simulink model "Mounna_FrottementsNew"  (R2025b)
settings: Solver=ode45  StartTime=0.0  StopTime=TimeTqStop  MaxStep=0.1  RelTol=1e-3  EnableMultiTasking=on
undefined symbols (not defined in the file): Kv, RegimeTq, TempsTq, TorqueLosesTest, TorqueLosesTimeTest
settings Model: Creator=a030141  LastModifiedBy=Etudiant
settings SolverCC: AlgebraicLoopSolver=TrustRegion
settings DataIOCC: LimitDataPoints=on  SaveFormat=Array  SignalLoggingSaveFormat=ModelDataLogs  ReturnWorkspaceOutputs=off  SignalLoggingName=sigsOut
settings OptimizationCC: InitFltsAndDblsToZero=on  LifeSpan=inf
settings DebuggingCC: SaveWithParameterizedLinksMsg=none  UnderspecifiedInitializationDetection=Classic  MergeDetectMultiDrivingBlocksExec=none  SignalResolutionControl=TryResolveAllWithWarning  MultiTaskDSMMsg=warning  MultiTaskCondExecSysMsg=none  FcnCallInpInsideContextMsg=warning  UnconnectedInputMsg=warning  UnconnectedOutputMsg=warning  UnconnectedLineMsg=warning  SFUnexpectedBacktrackingDiag=warning  SFNoUnconditionalDefaultTransitionDiag=warning  SFExecutionAtInitializationDiag=none  ArithmeticOperatorsInVariantConditions=warning
settings HardwareCC: ProdBitPerPointer=32.0  ProdBitPerSizeT=32.0  ProdBitPerPtrDiffT=32.0  ProdLargestAtomicFloat=None  ProdIntDivRoundTo=Undefined  ProdEndianess=Unspecified  ProdWordSize=32.0  ProdHWDeviceType=32-bit Generic  TargetUnknown=on
settings ModelReferenceCC: PropagateSignalLabelsOutOfModel=off
settings RTWCC: GPUComputeCapability=3.5
settings CodeAppCC: StateflowObjectComments=on
settings GRTTargetCC: TargetFcnLib=ansi_tfl_tmw.mat  TargetLangStandard=C89/C90 (ANSI)  CombineOutputUpdateFcns=off  GRTInterface=on
settings ConfigComp: CovMetricSettings=dw  CovSaveCumulativeToWorkspaceVar=on  CovSaveSingleToWorkspaceVar=on

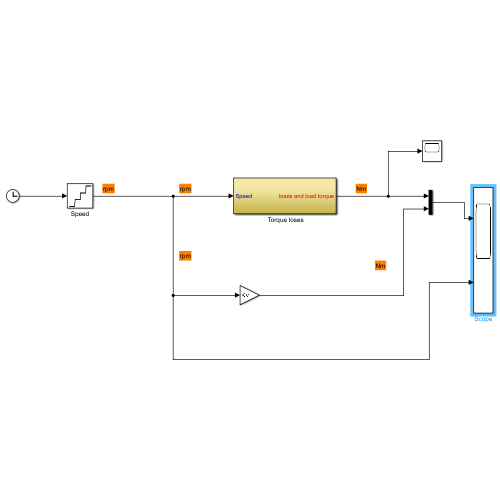
[thumbnail: Simulink's stored preview of the top-level diagram]
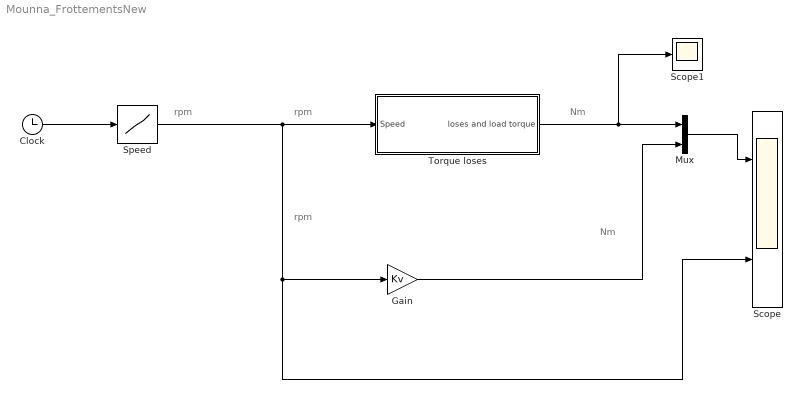
== system Mounna_FrottementsNew ==
  note: Nm
  note: rpm
  note: rpm
  note: rpm
  note: Nm
  " Torque loses" : Subsystem
  Clock : Clock
  Gain : Gain  Gain=Kv
  Mux : Mux  Inputs=2
  Scope : Scope  NumInputPorts=2
      settings: Title=Couple [Nm]  ActiveDisplayYMinimum=-114.2769674671385  ActiveDisplayYMaximum=10.919663051904275
  Scope1 : Scope
      settings: ActiveDisplayYMinimum=-1  ActiveDisplayYMaximum=1
  Speed : Lookup  InputValues=TempsTq  Table=RegimeTq
  wires:
  Clock/1 -> Speed/1
  Speed/1 -> Scope/2, Gain/1, " Torque loses"/1(Speed)
  Mux/1 -> Scope/1
  " Torque loses"/1(loses and load torque) -> Scope1/1, Mux/1
  Gain/1 -> Mux/2

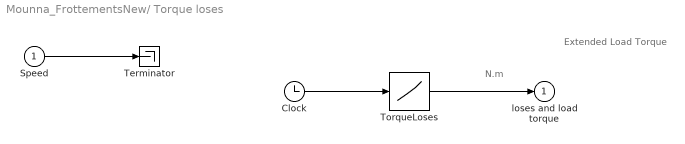
== system Mounna_FrottementsNew/ Torque loses ==
  note: N.m
  note: Extended Load Torque
  Speed : Inport
  Clock : Clock
  Terminator : Terminator
  TorqueLoses : Lookup  InputValues=TorqueLosesTimeTest  Table=TorqueLosesTest
  loses and load torque : Outport
  wires:
  Clock/1 -> TorqueLoses/1
  TorqueLoses/1 -> loses and load torque/1
  Speed/1 -> Terminator/1
